simulink model "GP_beta_saturation"  (R2022a)
settings: Solver=ode4  StartTime=0.0  StopTime=20  FixedStep=1e-3  RelTol=1e-3  EnableMultiTasking=on
values from neighbouring files (symbols this model uses):
  coeff_den_s = 2*par.kseta/par.w0    [GP_main_run.m]
  coeff_den_s2 = 1/par.w0^2    [GP_main_run.m]
  coeff_num_s = par.mass*par.l_f*V_ref/(par.L*par.Calpha_rear)    [GP_main_run.m]
  LQR_K = LQR_K'    [GP_main_run.m]
  LQR_Vx_ref = linspace(10,V_kmph,n_points)/3.6    [GP_main_run.m]
  V_ref = V_kmph /3.6    (= 27.7777777778)    [GP_main_run.m]
undefined symbols (not defined in the file or in its folder): par
libraries: simulink x2
settings Model: Creator=bshyrokau  LastModifiedBy=31682
settings SolverCC: AlgebraicLoopSolver=TrustRegion
settings DataIOCC: SaveOutput=off  SignalLogging=off  DSMLogging=off  SaveTime=off  ReturnWorkspaceOutputs=off
settings OptimizationCC: LifeSpan=inf
settings DebuggingCC: UnconnectedInputMsg=warning  UnconnectedOutputMsg=warning  UnconnectedLineMsg=warning  AllowSymbolicDim=off  SFUnexpectedBacktrackingDiag=warning  SFNoUnconditionalDefaultTransitionDiag=warning  SFExecutionAtInitializationDiag=none  SFMachineParentedDataDiag=warning  ArithmeticOperatorsInVariantConditions=warning
settings ModelReferenceCC: PropagateSignalLabelsOutOfModel=off
settings SFSimCC: SimUseLocalCustomCode=off  CustomCodeUndefinedFunction=UseInterfaceOnly
settings RTWCC: RTWUseLocalCustomCode=off  DLArmComputeVersion=19.05
settings CodeAppCC: StateflowObjectComments=on
settings GRTTargetCC: TargetLangStandard=C89/C90 (ANSI)
settings ConfigComp: CovMetricSettings=dw  CovSaveCumulativeToWorkspaceVar=on  CovSaveSingleToWorkspaceVar=on  CovExternalEMLEnable=off
settings SimscapeCC: SimscapeNormalizeSystem=off
settings ConfigurationSet: Description=SimMechanics 2G

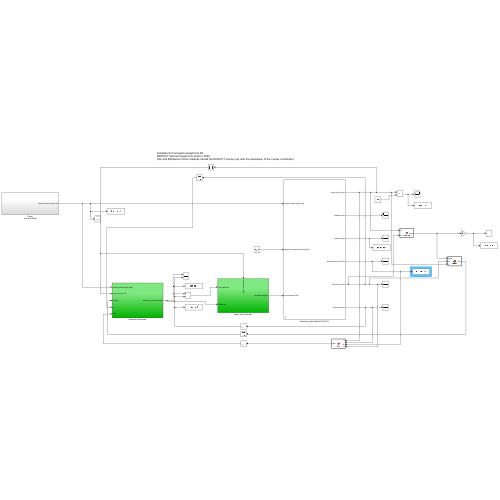
[thumbnail: Simulink's stored preview of the top-level diagram]
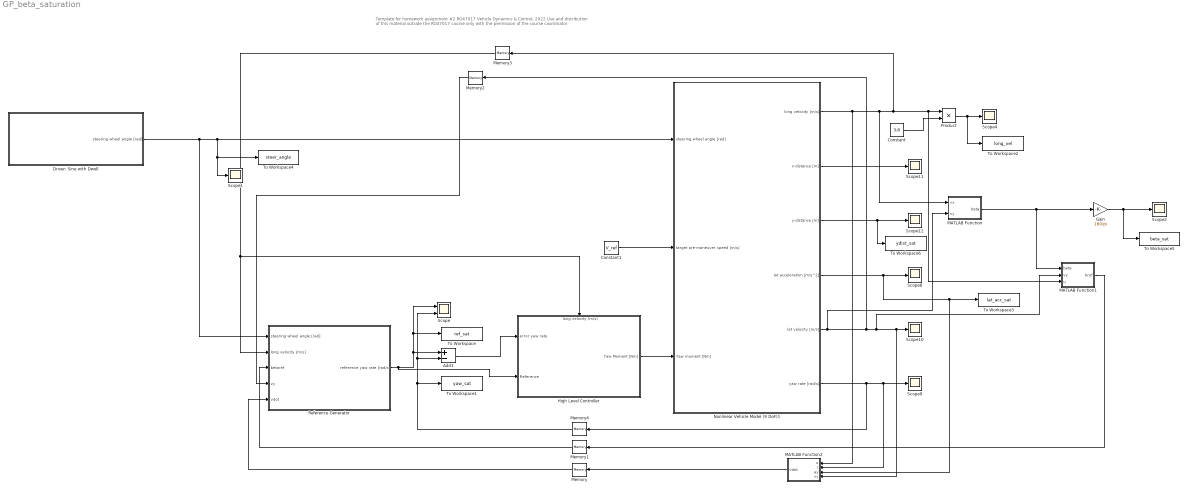
== system GP_beta_saturation ==
  note: Template for homework assignment #2
      | RO47017 Vehicle Dynamics & Control, 2022
      | Use and distribution of this material outside the RO47017 course only with the permission of the course coordinator
  Add1 : Sum  Inputs=+-
  Constant : Constant  Value=3.6
  Constant1 : Constant  Value=V_ref
  Driver: Sine with Dwell : Subsystem
  Gain : Gain  Gain=180/pi
  High Level Controller : Subsystem
      settings: PortSchema="{\"entries\":[{\"content\":{\"sides\":[{\"content\":{\"connectorIds\":[\"In1\",\"In2\"]},\"type\":\"ConnectorPlacement.EquallySpacedRectSide\",\"uuid\":\"b384b34b-9bc0-4dc4-b497-a1a499aa981c\"},{\"content\":{\"connectorIds\":[\"Out1\"],\"side\":\"RIGHT\"},\"type\":\"ConnectorPlacement.EquallySpacedRectSide\",\"uuid\":\"f3fdbba3-f0c8-4c56-b5d3-57c2637e329a\"},{\"content\":{\"connectorIds\":[\"In3\"],\"side\":\"TOP\"},\"type\":\"ConnectorPlacement.EquallySpacedRectSide\",\"uuid\":\"8207fb3d-652b-4ff7-8aca-b12b8e9d27cb\"}]},\"type\":\"ConnectorPlacement.EquallySpacedConnector\",\"uuid\":\"b3f519a7-c6c9-4b81-97c5-4685209ce260\"}],\"packageUris\":[\"http://schema.mathworks.com/mf0/Connector/R2020b\"],\"version\":\"1.0\"}"
  MATLAB Function : MATLAB Function  TreatAsAtomicUnit=on
  MATLAB Function1 : MATLAB Function  TreatAsAtomicUnit=on
  MATLAB Function2 : MATLAB Function  TreatAsAtomicUnit=on
  Memory{,1..4} (5 alike) : Memory
  Nonlinear Vehicle Model (9 DoF)1 : Subsystem
      mask help: Simulink:masks:GenSFuncDesc_MD
      mask Help: eval('feval(''rtwprivate'',''rtwhelpview'',''rtw_sfcn_block'')');
  Product : Product
  Reference Generator : Subsystem
  Scope : Scope  NumInputPorts=2
  Scope{1..2,4,8..12} (8 alike) : Scope
  To Workspace : ToWorkspace  VariableName=ref_sat  SaveFormat=Timeseries  SampleTime=-1
  To Workspace1 : ToWorkspace  VariableName=yaw_sat  SaveFormat=Timeseries  SampleTime=-1
  To Workspace2 : ToWorkspace  VariableName=long_vel  SaveFormat=Timeseries  SampleTime=-1
  To Workspace3 : ToWorkspace  VariableName=lat_acc_sat  SaveFormat=Timeseries  SampleTime=-1
  To Workspace4 : ToWorkspace  VariableName=steer_angle  SaveFormat=Timeseries  SampleTime=-1
  To Workspace5 : ToWorkspace  VariableName=beta_sat  SaveFormat=Timeseries  SampleTime=-1
  To Workspace6 : ToWorkspace  VariableName=ydist_sat  SaveFormat=Timeseries  SampleTime=-1
  wires:
  Nonlinear Vehicle Model (9 DoF)1/3(y-distance [m]) -> To Workspace6/1, Scope12/1
  Nonlinear Vehicle Model (9 DoF)1/4(lat acceleration [m/s^2]) -> MATLAB Function2/3(ay), To Workspace3/1, Scope8/1
  Driver: Sine with Dwell/1(steering wheel angle [rad]) -> To Workspace4/1, Scope1/1, Nonlinear Vehicle Model (9 DoF)1/1(steering wheel angle [rad]), Reference Generator/1(steering wheel angle [rad])
  Nonlinear Vehicle Model (9 DoF)1/2(x-distance [m]) -> Scope11/1
  Nonlinear Vehicle Model (9 DoF)1/6(yaw rate [rad/s]) -> MATLAB Function2/2(r), Scope9/1, Memory4/1
  Product/1 -> To Workspace2/1, Scope4/1
  High Level Controller/1(Yaw Moment [Nm]) -> Nonlinear Vehicle Model (9 DoF)1/3(Yaw moment [Nm])
  Constant/1 -> Product/2
  Constant1/1 -> Nonlinear Vehicle Model (9 DoF)1/2(target pre-maneuver speed [m/s])
  Add1/1 -> High Level Controller/1(error yaw rate)
  Gain/1 -> Scope2/1, To Workspace5/1
  Nonlinear Vehicle Model (9 DoF)1/5(lat velocity [m/s]) -> MATLAB Function/2(vy), Memory2/1, MATLAB Function1/2(vy), MATLAB Function2/4(vy), Scope10/1
  Nonlinear Vehicle Model (9 DoF)1/1(long velocity [m/s]) -> MATLAB Function2/1(u), MATLAB Function/1(vx), MATLAB Function1/3(u), Product/1, Memory3/1
  MATLAB Function/1(beta) -> Gain/1, MATLAB Function1/1(beta)
  MATLAB Function1/1(bref) -> Memory1/1
  MATLAB Function2/1(vdot) -> Memory/1
  Memory/1 -> Reference Generator/5(vdot)
  Memory1/1 -> Reference Generator/3(betaref)
  Memory2/1 -> Reference Generator/4(vy)
  Memory3/1 -> High Level Controller/3(long velocity (m/s)), Reference Generator/2(long velocity [m/s])
  Reference Generator/1(reference yaw rate [rad/s]) -> High Level Controller/2(Reference), Scope/1, To Workspace/1, Add1/1
  Memory4/1 -> To Workspace1/1, Scope/2, Add1/2

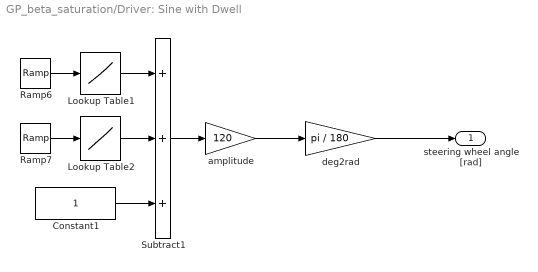
== system GP_beta_saturation/Driver: Sine with Dwell ==
  Constant1 : Constant
  Lookup Table1 : Lookup  InputValues=[0:0.1:3*pi/2 3*pi/2+eps]*0.7  Table=sin([0:0.1:3*pi/2 3*pi/2+eps])  LookUpMeth=Interpolation-Use End Values  SaturateOnIntegerOverflow=off
  Lookup Table2 : Lookup  InputValues=[3*pi/2:0.1:2*pi 2*pi+eps]*0.7  Table=sin([3*pi/2:0.1:2*pi 2*pi+eps])  LookUpMeth=Interpolation-Use End Values  SaturateOnIntegerOverflow=off
  Ramp6 : simulink/Sources/Ramp  slope=pi  start=10  InitialOutput=0
  Ramp7 : simulink/Sources/Ramp  slope=pi  start=10+0.5  InitialOutput=0
  Subtract1 : Sum  Inputs=+++
  amplitude : Gain  Gain=120
  deg2rad : Gain  Gain=pi / 180
  steering wheel angle [rad] : Outport  VectorParamsAs1DForOutWhenUnconnected=off
  wires:
  Ramp6/1 -> Lookup Table1/1
  Ramp7/1 -> Lookup Table2/1
  Lookup Table2/1 -> Subtract1/2
  Lookup Table1/1 -> Subtract1/1
  Constant1/1 -> Subtract1/3
  Subtract1/1 -> amplitude/1
  amplitude/1 -> deg2rad/1
  deg2rad/1 -> steering wheel angle [rad]/1

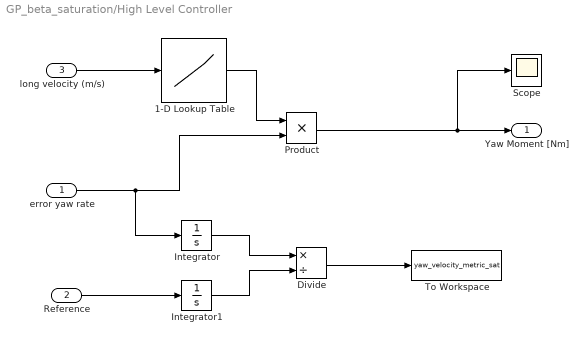
== system GP_beta_saturation/High Level Controller ==
  error yaw rate : Inport
  Reference : Inport  Port=2
  long velocity (m/s) : Inport  Port=3
  1-D Lookup Table : Lookup_n-D  NumberOfTableDimensions=1  BreakpointsForDimension1=LQR_Vx_ref  Table=LQR_K(2,:)  InternalRulePriority=Speed  RndMeth=Simplest
  Divide : Product  Inputs=*/
  Integrator : Integrator
  Integrator1 : Integrator
  Product : Product
  Scope : Scope
  To Workspace : ToWorkspace  VariableName=yaw_velocity_metric_sat  SaveFormat=Timeseries  SampleTime=-1
  Yaw Moment [Nm] : Outport  VectorParamsAs1DForOutWhenUnconnected=off
  wires:
  long velocity (m/s)/1 -> 1-D Lookup Table/1
  1-D Lookup Table/1 -> Product/1
  Product/1 -> Scope/1, Yaw Moment [Nm]/1
  Reference/1 -> Integrator1/1
  Divide/1 -> To Workspace/1
  Integrator/1 -> Divide/1
  Integrator1/1 -> Divide/2
  error yaw rate/1 -> Integrator/1, Product/2

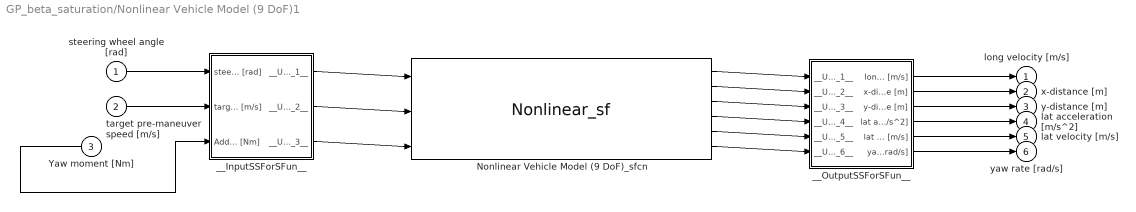
== system GP_beta_saturation/Nonlinear Vehicle Model (9 DoF)1 ==
  steering wheel angle [rad] : Inport
  target pre-maneuver speed [m/s] : Inport  Port=2
  Yaw moment [Nm] : Inport  Port=3
  Nonlinear Vehicle Model (9 DoF)_sfcn : S-Function  FunctionName=Nonlinear_sf  SFunctionModules=""  SFunctionDeploymentMode=off  EnableBusSupport=off  mask{rtw_sf_name=Nonlinear_sf, showVar=off}
      mask prompts: rtw_sf_name "Simulink:masks:GenSFuncName_MP"; showVar "Simulink:masks:GenSFuncShowModuleList_MP"
      mask help: Simulink:masks:GenSFuncDesc_MD
      mask init:
      | displist = '';
      | if ~strcmp(get_param(gcb, 'FunctionName'), rtw_sf_name);
      |   set_param(gcb, 'FunctionName', rtw_sf_name);
      | end
      | % Check if we are generating code
      | rtw_mode = false;
      | if strcmpi(get_param(bdroot(gcb),'SimulationStatus'),'Initializing')
      | 	rtw_mode = strcmpi(get_param(bdroot(gcb),'BuildingRTWCode'),'on') && ...
      | 		~strcmpi(get_param(bdroot(gcb),'TargetStyle'),'SimulationTarget');
      | end
      | if showVar || rtw_mode
      | 	if exist('rtwsfunc') == 2 | exist('rtwsfunc') == 6
      | 		tmplist = rtwsfunc(rtw_sf_name,gcb);
      | 		tmplist = DAStudio.message('Simulink:masks:GenSFuncListOfModules_IC', tmplist);
      | 	elseif showVar
      | 		tmplist1 = DAStudio.message('Simulink:masks:GenSFuncListOfModules_IC', '');
      |         tmplist2 = DAStudio.message('Simulink:masks:GenSFuncNotLicensed_IC');
      |         tmplist = [tmplist1 tmplist2];
      |  	end
      | end
      | if showVar
      |   displist = tmplist;
      | end
      settings: CopyFcn=|
      | if ~strcmp(get_param(gcb,'Linkstatus'),'none') && ...
      | ~strcmp(get_param(gcb,'Linkstatus'),'implicit')
      |   set_param(gcb,'LinkStatus','none');
      | end
      mask Help: eval('feval(''rtwprivate'',''rtwhelpview'',''rtw_sfcn_block'')');
      mask Display:
      | port_label('input',1,'steering wheel angle [rad]');
      | port_label('input',2,'target pre-maneuver speed [m/s]');
      | port_label('input',3,'Add yaw moment [Nm]');
      | port_label('output',1,'long velocity [m/s]');
      | port_label('output',2,'x-distance [m]');
      | port_label('output',3,'y-distance [m]');
      | port_label('output',4,'lat acceleration [m/s^2]');
      | port_label('output',5,'lat velocity [m/s]');
      | port_label('output',6,'yaw rate [rad/s]');
  __InputSSForSFun__ : Subsystem
  __OutputSSForSFun__ : Subsystem
  long velocity [m/s] : Outport  VectorParamsAs1DForOutWhenUnconnected=off
  x-distance [m] : Outport  Port=2  VectorParamsAs1DForOutWhenUnconnected=off
  y-distance [m] : Outport  Port=3  VectorParamsAs1DForOutWhenUnconnected=off
  lat acceleration [m/s^2] : Outport  Port=4  VectorParamsAs1DForOutWhenUnconnected=off
  lat velocity [m/s] : Outport  Port=5  VectorParamsAs1DForOutWhenUnconnected=off
  yaw rate [rad/s] : Outport  Port=6  VectorParamsAs1DForOutWhenUnconnected=off
  wires:
  steering wheel angle [rad]/1 -> __InputSSForSFun__/1(steering wheel angle [rad])
  target pre-maneuver speed [m/s]/1 -> __InputSSForSFun__/2(target pre-maneuver speed [m/s])
  Yaw moment [Nm]/1 -> __InputSSForSFun__/3(Add yaw moment [Nm])
  __InputSSForSFun__/1(__UniqueOutportName__1__) -> Nonlinear Vehicle Model (9 DoF)_sfcn/1
  __InputSSForSFun__/2(__UniqueOutportName__2__) -> Nonlinear Vehicle Model (9 DoF)_sfcn/2
  __InputSSForSFun__/3(__UniqueOutportName__3__) -> Nonlinear Vehicle Model (9 DoF)_sfcn/3
  Nonlinear Vehicle Model (9 DoF)_sfcn/1 -> __OutputSSForSFun__/1(__UniqueInportName__1__)
  Nonlinear Vehicle Model (9 DoF)_sfcn/2 -> __OutputSSForSFun__/2(__UniqueInportName__2__)
  Nonlinear Vehicle Model (9 DoF)_sfcn/3 -> __OutputSSForSFun__/3(__UniqueInportName__3__)
  Nonlinear Vehicle Model (9 DoF)_sfcn/4 -> __OutputSSForSFun__/4(__UniqueInportName__4__)
  Nonlinear Vehicle Model (9 DoF)_sfcn/5 -> __OutputSSForSFun__/5(__UniqueInportName__5__)
  Nonlinear Vehicle Model (9 DoF)_sfcn/6 -> __OutputSSForSFun__/6(__UniqueInportName__6__)
  __OutputSSForSFun__/1(long velocity [m/s]) -> long velocity [m/s]/1
  __OutputSSForSFun__/2(x-distance [m]) -> x-distance [m]/1
  __OutputSSForSFun__/3(y-distance [m]) -> y-distance [m]/1
  __OutputSSForSFun__/4(lat acceleration [m/s^2]) -> lat acceleration [m/s^2]/1
  __OutputSSForSFun__/5(lat velocity [m/s]) -> lat velocity [m/s]/1
  __OutputSSForSFun__/6(yaw rate [rad/s]) -> yaw rate [rad/s]/1

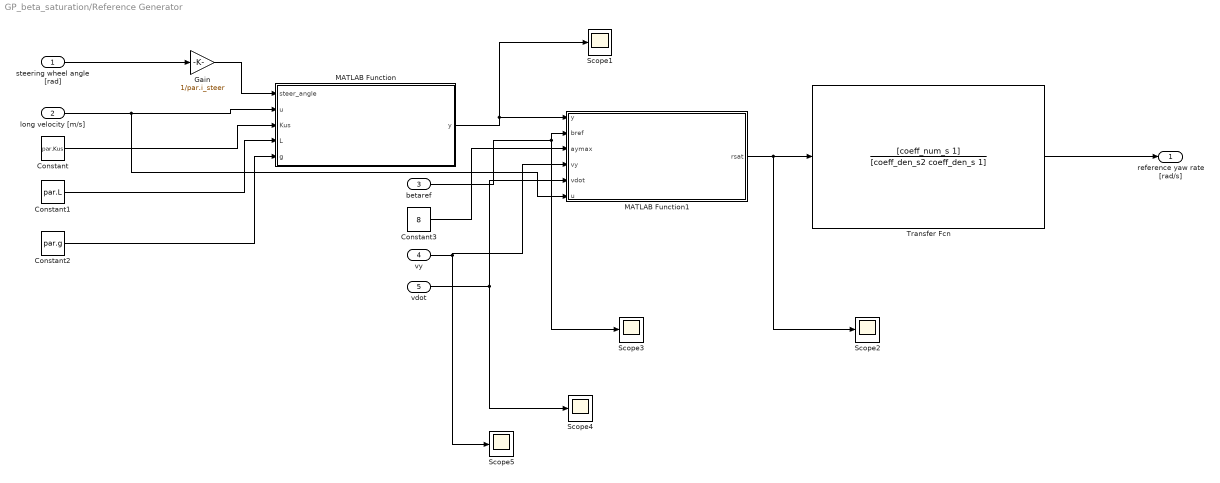
== system GP_beta_saturation/Reference Generator ==
  steering wheel angle [rad] : Inport
  long velocity [m/s] : Inport  Port=2
  betaref : Inport  Port=3
  vy : Inport  Port=4
  vdot : Inport  Port=5
  Constant : Constant  Value=par.Kus
  Constant1 : Constant  Value=par.L
  Constant2 : Constant  Value=par.g
  Constant3 : Constant  Value=8
  Gain : Gain  Gain=1/par.i_steer
  MATLAB Function : MATLAB Function  TreatAsAtomicUnit=on
  MATLAB Function1 : MATLAB Function  TreatAsAtomicUnit=on
  Scope{1..5} (5 alike) : Scope
  Transfer Fcn : TransferFcn  Numerator=[coeff_num_s 1]  Denominator=[coeff_den_s2 coeff_den_s 1]
  reference yaw rate [rad/s] : Outport  VectorParamsAs1DForOutWhenUnconnected=off
  wires:
  long velocity [m/s]/1 -> MATLAB Function1/6(u), MATLAB Function/2(u)
  Constant/1 -> MATLAB Function/3(Kus)
  Constant1/1 -> MATLAB Function/4(L)
  Constant2/1 -> MATLAB Function/5(g)
  Gain/1 -> MATLAB Function/1(steer_angle)
  steering wheel angle [rad]/1 -> Gain/1
  Transfer Fcn/1 -> reference yaw rate [rad/s]/1
  MATLAB Function/1(y) -> Scope1/1, MATLAB Function1/1(y)
  MATLAB Function1/1(rsat) -> Scope2/1, Transfer Fcn/1
  betaref/1 -> Scope3/1, MATLAB Function1/2(bref)
  Constant3/1 -> MATLAB Function1/3(aymax)
  vy/1 -> Scope5/1, MATLAB Function1/4(vy)
  vdot/1 -> Scope4/1, MATLAB Function1/5(vdot)

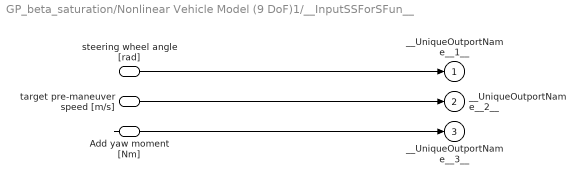
== system GP_beta_saturation/Nonlinear Vehicle Model (9 DoF)1/__InputSSForSFun__ ==
  steering wheel angle [rad] : Inport
  target pre-maneuver speed [m/s] : Inport  Port=2
  Add yaw moment [Nm] : Inport  Port=3
  __UniqueOutportName__1__ : Outport
  __UniqueOutportName__2__ : Outport  Port=2
  __UniqueOutportName__3__ : Outport  Port=3
  wires:
  steering wheel angle [rad]/1 -> __UniqueOutportName__1__/1
  target pre-maneuver speed [m/s]/1 -> __UniqueOutportName__2__/1
  Add yaw moment [Nm]/1 -> __UniqueOutportName__3__/1

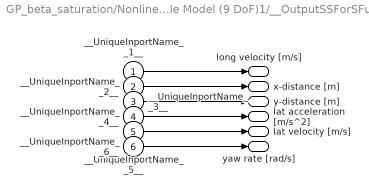
== system GP_beta_saturation/Nonlinear Vehicle Model (9 DoF)1/__OutputSSForSFun__ ==
  __UniqueInportName__1__ : Inport
  __UniqueInportName__2__ : Inport  Port=2
  __UniqueInportName__3__ : Inport  Port=3
  __UniqueInportName__4__ : Inport  Port=4
  __UniqueInportName__5__ : Inport  Port=5
  __UniqueInportName__6__ : Inport  Port=6
  long velocity [m/s] : Outport  VectorParamsAs1DForOutWhenUnconnected=off
  x-distance [m] : Outport  Port=2  VectorParamsAs1DForOutWhenUnconnected=off
  y-distance [m] : Outport  Port=3  VectorParamsAs1DForOutWhenUnconnected=off
  lat acceleration [m/s^2] : Outport  Port=4  VectorParamsAs1DForOutWhenUnconnected=off
  lat velocity [m/s] : Outport  Port=5  VectorParamsAs1DForOutWhenUnconnected=off
  yaw rate [rad/s] : Outport  Port=6  VectorParamsAs1DForOutWhenUnconnected=off
  wires:
  __UniqueInportName__1__/1 -> long velocity [m/s]/1
  __UniqueInportName__2__/1 -> x-distance [m]/1
  __UniqueInportName__3__/1 -> y-distance [m]/1
  __UniqueInportName__4__/1 -> lat acceleration [m/s^2]/1
  __UniqueInportName__5__/1 -> lat velocity [m/s]/1
  __UniqueInportName__6__/1 -> yaw rate [rad/s]/1

== matlab function GP_beta_saturation/Reference Generator/MATLAB Function ==
  data: steer_angle input; u input; y output; Kus input; L input; g input
function y = fcn(steer_angle, u, Kus, L, g)
    y = ( u / (L + ((Kus * u * u) / g ))) * steer_angle;
end

== matlab function GP_beta_saturation/Reference Generator/MATLAB Function1 ==
  data: y input; rsat output; bref input; aymax input; vy input; vdot input; u input
function rsat = aylimiter(y, bref,aymax,vy,vdot,u)
    ymax = (aymax - vdot*sin(bref))/(sqrt(u^2 + vy^2)*cos(bref));
    if(abs(y)<=ymax)
        rsat = y;
    else
        rsat = ymax*sign(y);
    end 
end

== matlab function GP_beta_saturation/MATLAB Function ==
  data: vx input; beta output; vy input
function beta = sideslip(vx,vy)

beta = atan(vy/vx);

end

== matlab function GP_beta_saturation/MATLAB Function1 ==
  data: beta input; bref output; vy input; u input
function bref = bmax(beta,vy,u)
vcog2 = vy^2 + u^2;
betamax = (10 - ((7*vcog2)/(1600)))*pi/180;

if(abs(beta)<=abs(betamax))
    bref = beta;
else
    bref = betamax*sign(beta);
end
end

== matlab function GP_beta_saturation/MATLAB Function2 ==
  data: u input; vdot output; r input; ay input; vy input
function vdot = fcn(u,r,ay,vy)

vcog2 = u^2 + vy^2;
vdot = vcog2^(-0.5)*vy*(ay-u*r);

end
